simulink model "case3_16AE10005"  (R2017b)
settings: Solver=ode4  StartTime=0.0  StopTime=50  FixedStep=0.0001  RelTol=1e-3
libraries: simulink x5
settings Model: Creator=ayushi  LastModifiedBy=ayushi

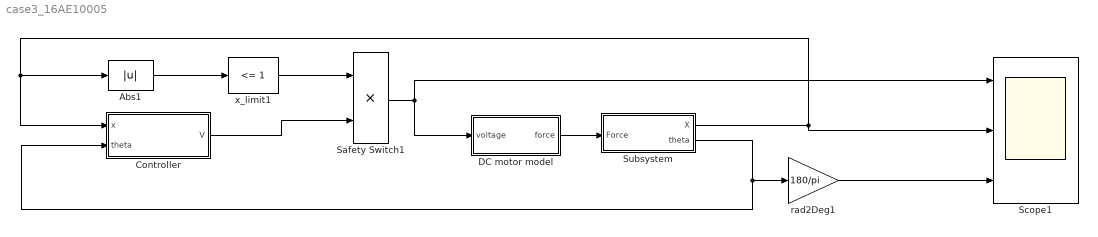
== system case3_16AE10005 ==
  Abs1 : Abs
  "Controller " : Subsystem
  DC motor model : Subsystem
  Safety Switch1 : Product
  Scope1 : Scope  NumInputPorts=3
  Subsystem : Subsystem
  rad2Deg1 : Gain  Gain=180/pi
  x_limit1 : simulink/Logic and Bit Operations/Compare To Constant  relop=<=  const=1  OutDataTypeStr=boolean
  wires:
  rad2Deg1/1 -> Scope1/3
  Safety Switch1/1 -> DC motor model/1(voltage), Scope1/1
  Subsystem/2("theta ") -> "Controller "/2(theta), rad2Deg1/1
  "Controller "/1(V) -> Safety Switch1/2
  Abs1/1 -> x_limit1/1
  Subsystem/1("X ") -> Scope1/2, "Controller "/1(x), Abs1/1
  DC motor model/1(force) -> Subsystem/1(Force)
  x_limit1/1 -> Safety Switch1/1

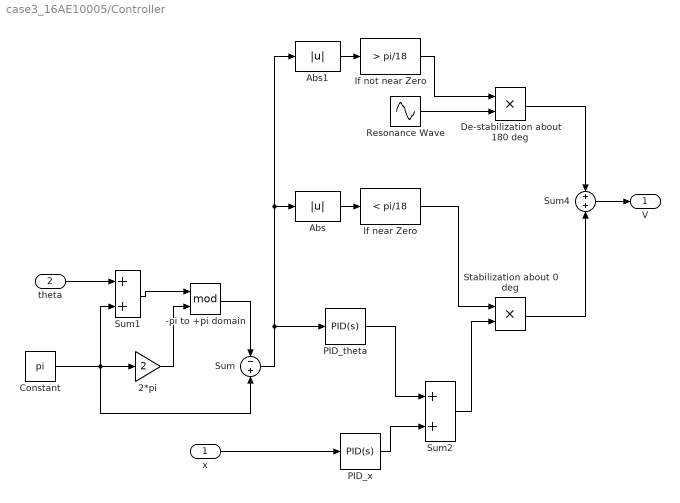
== system case3_16AE10005/Controller  ==
  x : Inport
  theta : Inport  Port=2
  -pi to +pi domain : Math  Operator=mod  SaturateOnIntegerOverflow=on
  2*pi : Gain  Gain=2
  Abs : Abs  RndMeth=Nearest
  Abs1 : Abs
  Constant : Constant  Value=pi
  De-stabilization about 180 deg : Product
  If near Zero : simulink/Logic and Bit Operations/Compare To Constant  relop=<  const=pi/18  OutDataTypeStr=boolean
  If not near Zero : simulink/Logic and Bit Operations/Compare To Constant  relop=>  const=pi/18  OutDataTypeStr=boolean
  PID_theta : simulink/Continuous/PID Controller  Controller=PID  TimeDomain=Continuous-time  SampleTime=-1  IntegratorMethod=Forward Euler  FilterMethod=Forward Euler  Form=Parallel  UseFilter=on  ControllerParametersSource=internal  P=25  I=2  D=50  N=1000  InitialConditionSource=internal  InitialConditionForIntegrator=0  InitialConditionForFilter=0  ExternalReset=none  LimitOutput=off  UpperSaturationLimit=inf  LowerSaturationLimit=-inf  LinearizeAsGain=on  AntiWindupMode=none  Kb=1  TrackingMode=off  Kt=1  PParamMin=[]  PParamMax=[]  IParamMin=[]  IParamMax=[]  DParamMin=[]  DParamMax=[]  NParamMin=[]  NParamMax=[]  KbParamMin=[]  KbParamMax=[]  KtParamMin=[]  KtParamMax=[]  POutMin=[]  POutMax=[]  IOutMin=[]  IOutMax=[]  DOutMin=[]  DOutMax=[]  NOutMin=[]  NOutMax=[]  KbOutMin=[]  KbOutMax=[]  KtOutMin=[]  KtOutMax=[]  IntegratorOutMin=[]  IntegratorOutMax=[]  FilterOutMin=[]  FilterOutMax=[]  SumOutMin=[]  SumOutMax=[]  SumI1OutMin=[]  SumI1OutMax=[]  SumI2OutMin=[]  SumI2OutMax=[]  SumI3OutMin=[]  SumI3OutMax=[]  SumDOutMin=[]  SumDOutMax=[]  SaturationOutMin=[]  SaturationOutMax=[]  IntegratorContinuousStateAttributes=''  IntegratorStateMustResolveToSignalObject=off  IntegratorRTWStateStorageClass=Auto  FilterContinuousStateAttributes=''  FilterStateMustResolveToSignalObject=off  FilterRTWStateStorageClass=Auto  DifferentiatorICPrevScaledInput=0  DifferentiatorOutMin=[]  DifferentiatorOutMax=[]  InitialConditionSetting=State (most efficient)  FilterDiffOutCoefMin=[]  FilterDiffOutCoefMax=[]  SumDenOutMin=[]  SumDenOutMax=[]  SumNumOutMin=[]  SumNumOutMax=[]  ReciprocalOutMin=[]  ReciprocalOutMax=[]  DivideOutMin=[]  DivideOutMax=[]  TunerSelectOption=Transfer Function Based (PID Tuner App)
  PID_x : simulink/Continuous/PID Controller  Controller=PID  TimeDomain=Continuous-time  SampleTime=-1  IntegratorMethod=Forward Euler  FilterMethod=Forward Euler  Form=Parallel  UseFilter=on  ControllerParametersSource=internal  P=30  I=4  D=0  N=1000  InitialConditionSource=internal  InitialConditionForIntegrator=0  InitialConditionForFilter=0  ExternalReset=none  LimitOutput=off  UpperSaturationLimit=inf  LowerSaturationLimit=-inf  LinearizeAsGain=on  AntiWindupMode=none  Kb=1  TrackingMode=off  Kt=1  PParamMin=[]  PParamMax=[]  IParamMin=[]  IParamMax=[]  DParamMin=[]  DParamMax=[]  NParamMin=[]  NParamMax=[]  KbParamMin=[]  KbParamMax=[]  KtParamMin=[]  KtParamMax=[]  POutMin=[]  POutMax=[]  IOutMin=[]  IOutMax=[]  DOutMin=[]  DOutMax=[]  NOutMin=[]  NOutMax=[]  KbOutMin=[]  KbOutMax=[]  KtOutMin=[]  KtOutMax=[]  IntegratorOutMin=[]  IntegratorOutMax=[]  FilterOutMin=[]  FilterOutMax=[]  SumOutMin=[]  SumOutMax=[]  SumI1OutMin=[]  SumI1OutMax=[]  SumI2OutMin=[]  SumI2OutMax=[]  SumI3OutMin=[]  SumI3OutMax=[]  SumDOutMin=[]  SumDOutMax=[]  SaturationOutMin=[]  SaturationOutMax=[]  IntegratorContinuousStateAttributes=''  IntegratorStateMustResolveToSignalObject=off  IntegratorRTWStateStorageClass=Auto  FilterContinuousStateAttributes=''  FilterStateMustResolveToSignalObject=off  FilterRTWStateStorageClass=Auto  DifferentiatorICPrevScaledInput=0  DifferentiatorOutMin=[]  DifferentiatorOutMax=[]  InitialConditionSetting=State (most efficient)  FilterDiffOutCoefMin=[]  FilterDiffOutCoefMax=[]  SumDenOutMin=[]  SumDenOutMax=[]  SumNumOutMin=[]  SumNumOutMax=[]  ReciprocalOutMin=[]  ReciprocalOutMax=[]  DivideOutMin=[]  DivideOutMax=[]  TunerSelectOption=Transfer Function Based (PID Tuner App)
  Resonance Wave : Sin  Amplitude=1.73  Frequency=2.2  Phase=pi/2  SampleTime=0
  Stabilization about 0 deg : Product
  Sum : Sum  Inputs=-+
  Sum1 : Sum
  Sum2 : Sum
  Sum4 : Sum
  V : Outport
  wires:
  Constant/1 -> Sum/2, 2*pi/1, Sum1/2
  theta/1 -> Sum1/1
  2*pi/1 -> -pi to +pi domain/2
  -pi to +pi domain/1 -> Sum/1
  Sum/1 -> PID_theta/1, Abs1/1, Abs/1
  Sum1/1 -> -pi to +pi domain/1
  If not near Zero/1 -> De-stabilization about 180 deg/1
  Sum4/1 -> V/1
  De-stabilization about 180 deg/1 -> Sum4/1
  Stabilization about 0 deg/1 -> Sum4/2
  Abs/1 -> If near Zero/1
  Abs1/1 -> If not near Zero/1
  Sum2/1 -> Stabilization about 0 deg/2
  If near Zero/1 -> Stabilization about 0 deg/1
  x/1 -> PID_x/1
  Resonance Wave/1 -> De-stabilization about 180 deg/2
  PID_theta/1 -> Sum2/1
  PID_x/1 -> Sum2/2

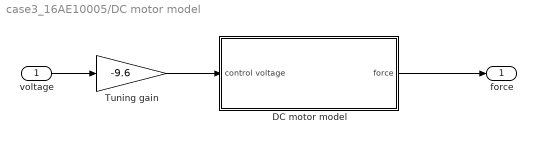
== system case3_16AE10005/DC motor model ==
  voltage : Inport
  DC motor model : Subsystem  mask{J=0.0000140, Kt=0.05, Kb=0.05, d=0.000001, R=2.5, L=0.0025}
      mask prompts: J "Moment of inertia"; Kt "Torque constant"; Kb "Electromotive force constant"; d "Linear approximation of viscous friction"; R "Electrical circuit resistance"; L "Electrical circuit inductance"
      mask Display: disp('DC motor')
  Tuning gain : Gain  Gain=-9.6
  force : Outport
  wires:
  Tuning gain/1 -> DC motor model/1(control voltage)
  voltage/1 -> Tuning gain/1
  DC motor model/1(force) -> force/1

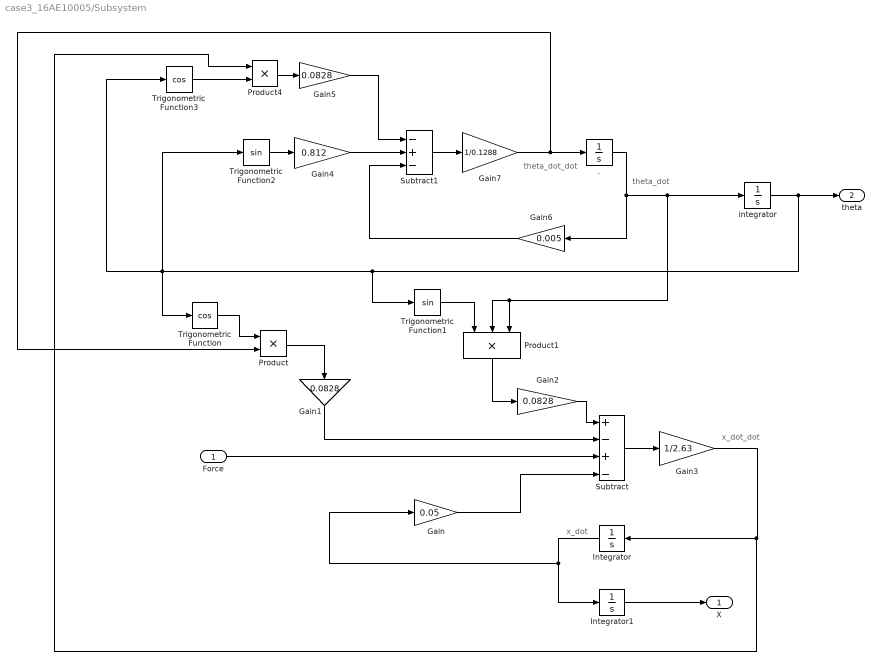
== system case3_16AE10005/Subsystem ==
  note: theta_dot
  note: theta_dot_dot
  note: x_dot
  note: x_dot_dot
  Force : Inport
  ". " : Integrator
  Gain : Gain  Gain=0.05
  Gain1 : Gain  Gain=0.0828
  Gain2 : Gain  Gain=0.0828
  Gain3 : Gain  Gain=1/2.63
  Gain4 : Gain  Gain=0.812
  Gain5 : Gain  Gain=0.0828
  Gain6 : Gain  Gain=0.005
  Gain7 : Gain  Gain=1/0.1288
  Integrator : Integrator
  Integrator1 : Integrator
  Product : Product
  Product1 : Product  Inputs=3
  Product4 : Product
  Subtract : Sum  Inputs=+-+-
  Subtract1 : Sum  Inputs=-+-
  Trigonometric Function : Trigonometry  Operator=cos
  Trigonometric Function1 : Trigonometry
  Trigonometric Function2 : Trigonometry
  Trigonometric Function3 : Trigonometry  Operator=cos
  integrator : Integrator
  "X " : Outport
  "theta " : Outport  Port=2
  wires:
  Trigonometric Function2/1 -> Gain4/1
  Integrator1/1 -> "X "/1
  integrator/1 -> "theta "/1, Trigonometric Function1/1, Trigonometric Function3/1, Trigonometric Function/1, Trigonometric Function2/1
  Gain/1 -> Subtract/4
  Integrator/1 -> Gain/1, Integrator1/1
  Gain3/1 -> Integrator/1, Product4/1
  Gain7/1 -> Product/2, ". "/1
  Product/1 -> Gain1/1
  Gain4/1 -> Subtract1/2
  Force/1 -> Subtract/3
  Product4/1 -> Gain5/1
  Trigonometric Function/1 -> Product/1
  Trigonometric Function1/1 -> Product1/1
  Trigonometric Function3/1 -> Product4/2
  Gain6/1 -> Subtract1/3
  ". "/1 -> Gain6/1, Product1/3, Product1/2, integrator/1
  Product1/1 -> Gain2/1
  Gain2/1 -> Subtract/1
  Gain1/1 -> Subtract/2
  Gain5/1 -> Subtract1/1
  Subtract/1 -> Gain3/1
  Subtract1/1 -> Gain7/1

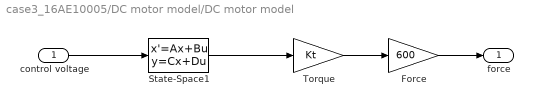
== system case3_16AE10005/DC motor model/DC motor model ==
  control voltage : Inport
  Force : Gain  Gain=600
  State-Space1 : StateSpace  A=[-d/J Kt/J;-Kb/L -R/L]  B=[0; 1/L]  C=[0 1]  D=0  InitialCondition=0
  Torque : Gain  Gain=Kt
  force : Outport
  wires:
  control voltage/1 -> State-Space1/1
  State-Space1/1 -> Torque/1
  Torque/1 -> Force/1
  Force/1 -> force/1
